simulink model "test01"  (R2021b)
settings: Solver=VariableStepAuto  StartTime=0.0  StopTime=10.0  RelTol=1e-3
settings Model: Creator=duanlinding  LastModifiedBy=duanlinding

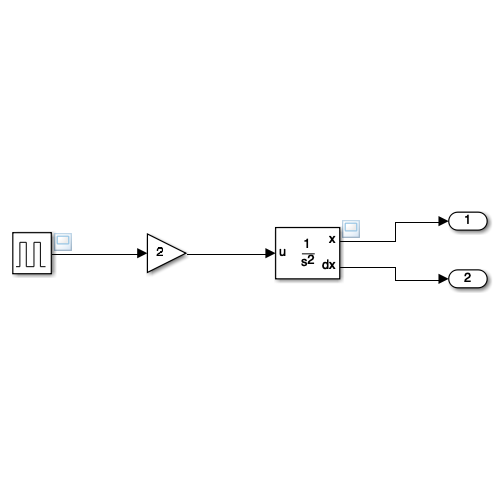
[thumbnail: Simulink's stored preview of the top-level diagram]
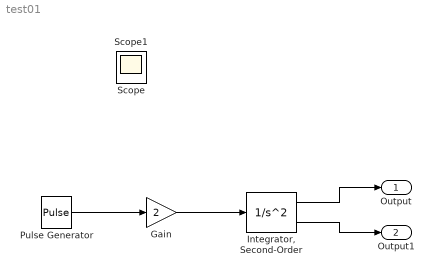
== system test01 ==
  Gain : Gain  Gain=2
  "Integrator, Second-Order" : SecondOrderIntegrator
  Pulse Generator : DiscretePulseGenerator  PulseType=Time based  Period=10  PulseWidth=5
  Output : Outport
  Output1 : Outport  Port=2
  Scope : Scope
  Scope1 : Scope
  wires:
  Pulse Generator/1 -> Gain/1
  Gain/1 -> "Integrator, Second-Order"/1
  "Integrator, Second-Order"/1 -> Output/1
  "Integrator, Second-Order"/2 -> Output1/1
